simulink model "rtwdemo_condinput"  (Simulink 6.0)
settings: Solver=FixedStepDiscrete  StartTime=0.0  StopTime=500  RelTol=1e-3
libraries: rtwdemowidgets x2
settings Model: Creator=The MathWorks Inc.  LastModifiedBy=batserve  ExtModeAutoUpdateStatusClock=off
settings DataIOCC: SaveOutput=off  SaveTime=off  SignalLoggingName=sigsOut
settings OptimizationCC: InlineParams=on  EnforceIntegerDowncast=off  StateBitsets=on  DataBitsets=on  UseTempVars=on
settings DebuggingCC: CheckExecutionContextPreStartOutputMsg=on  CheckExecutionContextRuntimeOutputMsg=on  SolverPrmCheckMsg=none
settings RTWCC: TLCOptions=-p0 -aWarnNonSaturatedBlocks=0  GenerateReport=on  RTWVerbose=off  ProcessScript=grt_make_rtw_hook  LaunchReport=on
settings CodeAppCC: ForceParamTrailComments=on  PrefixModelToSubsysFcnNames=off
settings GRTTargetCC: MatFileLogging=off

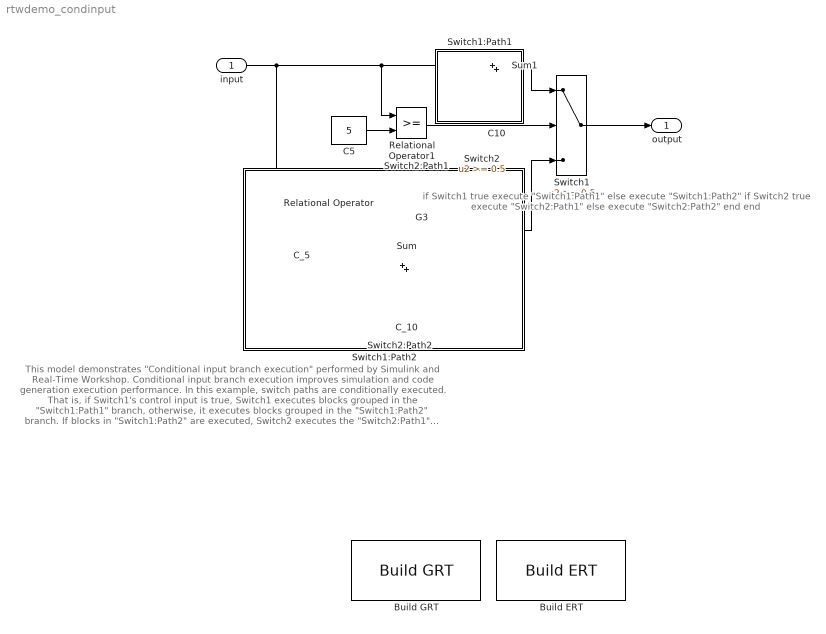
== system rtwdemo_condinput ==
  note: if Switch1 true
      |    execute "Switch1:Path1"
      |  else
      |    execute "Switch1:Path2"
      |    if Switch2 true
      |      execute "Switch2:Path1"
      |    else
      |      execute "Switch2:Path2"
      |    end
      |  end
  note: This model demonstrates "Conditional input branch execution" performed by Simulink and
      | Real-Time Workshop. Conditional input branch execution improves simulation and code
      | generation execution performance. In this example, switch paths are conditionally executed.
      | That is, if Switch1's control input is true, Switch1 executes blocks grouped in the
      | "Switch1:Path1" branch, otherwise, it executes blocks grouped in the "Switch1:Path2" branch.
      | If blocks in "Switch1:Path2" are executed, Switch2 executes the "Switch2:Path1" branch if
      | its control input is true.  Otherwise, it executes the "Switch2:Path2" branch.  This logic
      | is illustrated by the pseudo code above.
  input : Inport  Port=1  LatchInput=off
  "  C10" : Constant  Orientation=up  Value=10
  "  G3" : Gain  Gain=3  SaturateOnIntegerOverflow=on
  " C_10" : Constant  Orientation=up  Value=-10
  " Sum" : Sum  Inputs=|++  SaturateOnIntegerOverflow=on  InputSameDT=on
  " Sum1" : Sum  Inputs=|++  SaturateOnIntegerOverflow=on  InputSameDT=on
  " Switch2" : Switch  Threshold=0.5  SaturateOnIntegerOverflow=on  InputSameDT=on
  " Switch2:Path1" : Subsystem  Orientation=left  PropExecContextAcrossSSBoundary=on
      settings: AttributesFormatString=\n  OpenFcn=disp('');
      mask Display: disp(' ')
  " Switch2:Path2" : Subsystem  Orientation=left  PropExecContextAcrossSSBoundary=on
      settings: AttributesFormatString=\n  OpenFcn=disp('');
      mask Display: disp(' ')
  Build ERT : rtwdemowidgets/Build ERT  attrib_overrides={}
  Build GRT : rtwdemowidgets/Build GRT  attrib_overrides={}
  C5 : Constant  Value=5
  C_5 : Constant  Value=-5
  Relational Operator : RelationalOperator  InputSameDT=on
  Relational Operator1 : RelationalOperator  InputSameDT=on
  Switch1 : Switch  Threshold=0.5  SaturateOnIntegerOverflow=on  InputSameDT=on
  Switch1:Path1 : Subsystem  Orientation=left  PropExecContextAcrossSSBoundary=on
      settings: AttributesFormatString=\n  OpenFcn=disp('');
      mask Display: disp(' ')
  Switch1:Path2 : Subsystem  Orientation=left  PropExecContextAcrossSSBoundary=on
      settings: AttributesFormatString=\n  OpenFcn=disp('');
      mask Display: disp(' ')
  output : Outport
  wires:
  Relational Operator/1 -> " Switch2"/2
  " Switch2"/1 -> Switch1/3
  input/1 -> " Sum"/1, Relational Operator/1, "  G3"/1, Relational Operator1/1, " Sum1"/1
  "  G3"/1 -> " Switch2"/1
  " Sum1"/1 -> Switch1/1
  " Sum"/1 -> " Switch2"/3
  C5/1 -> Relational Operator1/2
  C_5/1 -> Relational Operator/2
  Switch1/1 -> output/1
  " C_10"/1 -> " Sum"/2
  "  C10"/1 -> " Sum1"/2
  Relational Operator1/1 -> Switch1/2

== system rtwdemo_condinput/ Switch2:Path1 ==

== system rtwdemo_condinput/ Switch2:Path2 ==

== system rtwdemo_condinput/Switch1:Path1 ==

== system rtwdemo_condinput/Switch1:Path2 ==
